simulink model "MainControl_v2"  (R2025a)
settings: Solver=ode45  StartTime=0.0  StopTime=inf  FixedStep=.1  RelTol=1e-3
undefined symbols (not defined in the file or in its folder): CR, DiscIntNeverNeededParam, LF
libraries: instrumentseriallib x3, simulink x1, dspstat3 x1
settings Model: PacingRate=1000  Creator=aceve  LastModifiedBy=diego

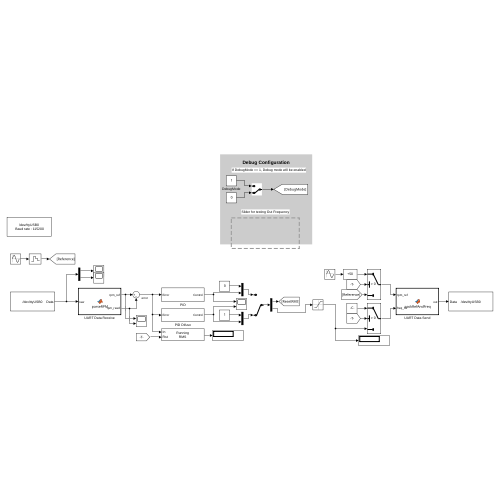
[thumbnail: Simulink's stored preview of the top-level diagram]
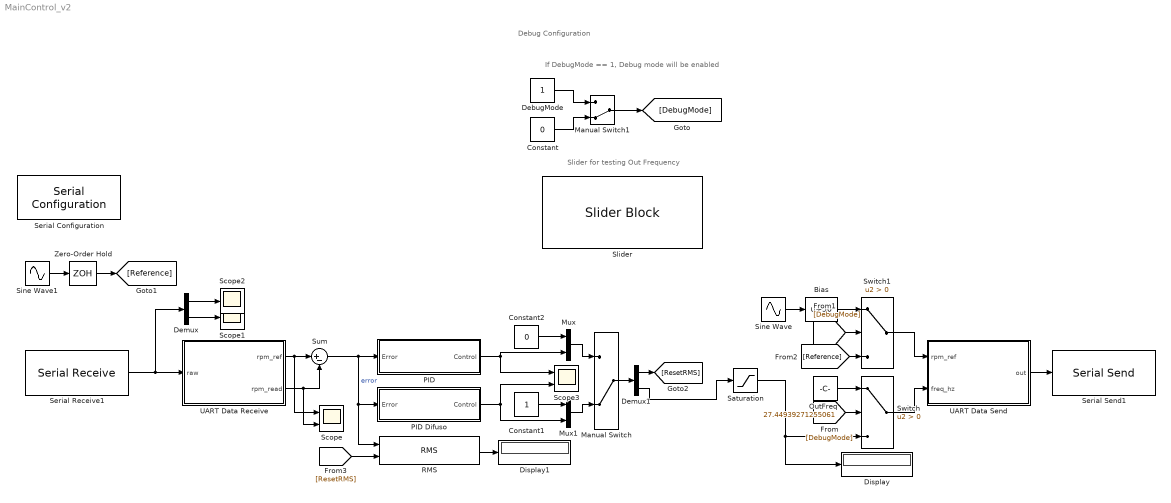
== system MainControl_v2 ==
  note: Debug Configuration
  note: If DebugMode == 1, Debug mode will be enabled
  note: Slider for testing Out Frequency
  Bias : Bias  Bias=50  SaturateOnIntegerOverflow=off
  Constant : Constant  Value=0
  Constant1 : Constant
  Constant2 : Constant  Value=0
  DebugMode : Constant
  Demux : Demux  Outputs=2
  Demux1 : Demux  Outputs=2
  Display : Display
  Display1 : Display
  Manual Switch : ManualSwitch  CurrentSetting=0
  Manual Switch1 : ManualSwitch  CurrentSetting=0
  Mux : Mux  Inputs=2
  Mux1 : Mux  Inputs=2
  OutFreq : Constant  Value=27.44939271255061
  PID : Subsystem
  PID Difuso : Subsystem
  RMS : dspstat3/RMS  run=on  directionMode=Entire input  dimension=1  InputProcessing=Columns as channels (frame based)  reset_popup=Either edge
  Saturation : Saturate  UpperLimit=60  LowerLimit=20
  Scope : Scope  NumInputPorts=2
      settings: ActiveDisplayYMinimum=-88.124999999999986  ActiveDisplayYMaximum=783.125
  Scope1 : Scope
      settings: ActiveDisplayYMinimum=-12.499999999999996  ActiveDisplayYMaximum=112.5
  Scope2 : Scope
      settings: ActiveDisplayYMinimum=-105.87499999999997  ActiveDisplayYMaximum=952.875  DataLoggingVariableName=ScopeData2
  Scope3 : Scope  NumInputPorts=2
      settings: ActiveDisplayYMinimum=-7.4999999999999982  ActiveDisplayYMaximum=67.5  DataLoggingVariableName=ScopeData3
  Serial Configuration : instrumentseriallib/Serial Configuration  Priority=-200000  PortSel=/dev/ttyUSB0  Port=/dev/ttyUSB0  ComPort=/dev/ttyUSB0  BaudRate=115200  DataBits=8  Parity=none  StopBits=1  ByteOrder=little-endian  FlowControl=none  Timeout=10  SimulateUsing=Interpreted execution  BlockInModel=on  aMode=1
  Serial Receive1 : instrumentseriallib/Serial Receive  Priority=1  PortSel=/dev/ttyUSB0  Port=/dev/ttyUSB0  ComPort=/dev/ttyUSB0  DataType=int16  SaveDataType=uint8  ToggleHeader=off  Header=[]  ToggleDataSize=on  DataSize=[2 1]  ToggleTerminator=off  Terminator=CR/LF ('\r\n')  CustomTerminator=[]  InputFormat=Column major  EnableBlockingMode=on  ActionDataUnavailable=Output last received value  ActionWhenDataUnavailable=Output last received value  CustomValue=0  SampleTime=0.01  SimulateUsing=Interpreted execution  BlockInModel=on  aMode=1  LibraryInUse=instrumentlib
  Serial Send1 : instrumentseriallib/Serial Send  Priority=1  PortSel=/dev/ttyUSB0  Port=/dev/ttyUSB0  ComPort=/dev/ttyUSB0  Header=[]  Terminator=<none>  CustomTerminator=[]  EnableBlockingMode=off  SimulateUsing=Interpreted execution  BlockInModel=on  aMode=1
  Sine Wave : Sin  Amplitude=50  SampleTime=0
  Sine Wave1 : Sin  Amplitude=20  Bias=500  Frequency=2  SampleTime=0
  Slider : SliderBlock  ScaleMin=20  ScaleMax=60
  Sum : Sum  Inputs=|+-
  Switch : Switch  Criteria=u2 > Threshold  SaturateOnIntegerOverflow=off  InputSameDT=off
  Switch1 : Switch  Criteria=u2 > Threshold  SaturateOnIntegerOverflow=off  InputSameDT=off
  UART Data Receive : MATLAB Function  TreatAsAtomicUnit=on
  UART Data Send : MATLAB Function  TreatAsAtomicUnit=on
  Zero-Order Hold : ZeroOrderHold  SampleTime=-1
  wires:
  Serial Receive1/1 -> Demux/1, UART Data Receive/1(raw)
  Demux/1 -> Scope2/1
  Demux/2 -> Scope1/1
  Sine Wave/1 -> Bias/1
  UART Data Send/1(out) -> Serial Send1/1
  Switch/1 -> UART Data Send/2(freq_hz)
  [DebugMode] -> Switch/2
  OutFreq/1 -> Switch/1
  Switch1/1 -> UART Data Send/1(rpm_ref)
  Bias/1 -> Switch1/1
  [DebugMode] -> Switch1/2
  Sum/1 -> PID Difuso/1(Error), RMS/1, PID/1(Error)  "error"
  PID Difuso/1(Control) -> Mux1/2, Scope3/2
  PID/1(Control) -> Mux/2, Scope3/1
  UART Data Receive/1(rpm_ref) -> Scope/1, Sum/1
  UART Data Receive/2(rpm_read) -> Scope/2, Sum/2
  Sine Wave1/1 -> Zero-Order Hold/1
  Zero-Order Hold/1 -> [Reference]
  [Reference] -> Switch1/3
  Saturation/1 -> Display/1, Switch/3
  DebugMode/1 -> Manual Switch1/1
  Manual Switch1/1 -> [DebugMode]
  Constant/1 -> Manual Switch1/2
  Constant1/1 -> Mux1/1
  Constant2/1 -> Mux/1
  Mux/1 -> Manual Switch/1
  Mux1/1 -> Manual Switch/2
  Manual Switch/1 -> Demux1/1
  Demux1/2 -> Saturation/1
  Demux1/1 -> [ResetRMS]
  [ResetRMS] -> RMS/2
  RMS/1 -> Display1/1

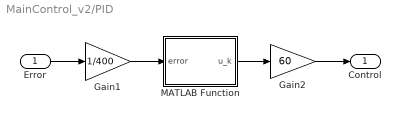
== system MainControl_v2/PID ==
  Error : Inport
  Gain1 : Gain  Gain=1/400
  Gain2 : Gain  Gain=60
  MATLAB Function : MATLAB Function  TreatAsAtomicUnit=on
  Control : Outport
  wires:
  Gain1/1 -> MATLAB Function/1(error)
  MATLAB Function/1(u_k) -> Gain2/1
  Error/1 -> Gain1/1
  Gain2/1 -> Control/1

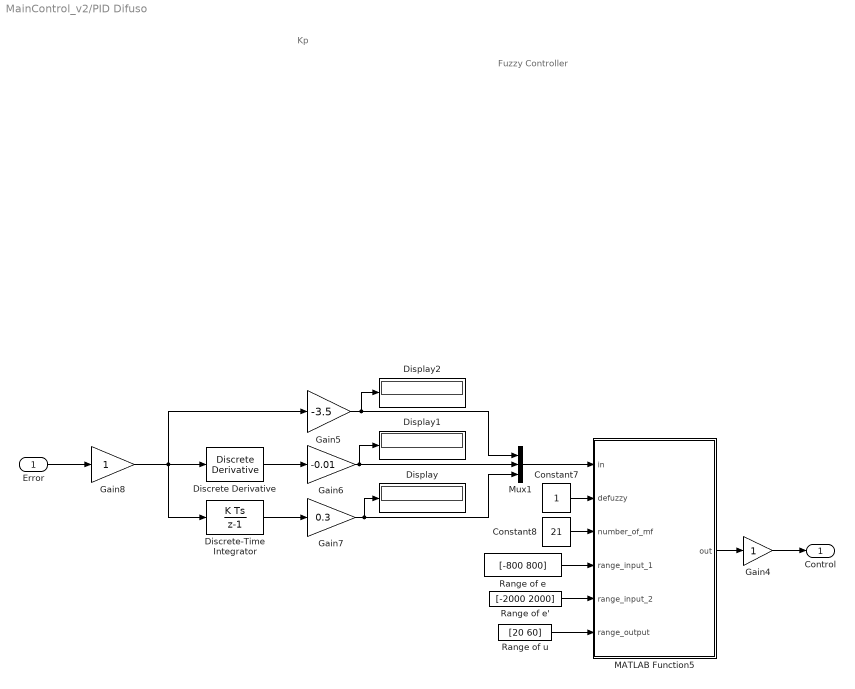
== system MainControl_v2/PID Difuso ==
  note: Fuzzy Controller
  note: Kp
  Error : Inport
  Constant7 : Constant
  Constant8 : Constant  Value=21
  Discrete Derivative : simulink/Discrete/Discrete Derivative  gainval=1.0  ICPrevScaledInput=0.0  OutMin=[]  OutMax=[]  OutDataType=fixdt(1, 16)  OutScaling=2^-10  DoSatur=off
  Discrete-Time Integrator : DiscreteIntegrator  InitialCondition=20  SampleTime=0.01  LimitOutput=on  UpperSaturationLimit=60  LowerSaturationLimit=-60  ICPrevOutput=DiscIntNeverNeededParam  ICPrevScaledInput=DiscIntNeverNeededParam
  Display : Display
  Display1 : Display
  Display2 : Display
  Gain4 : Gain
  Gain5 : Gain  Gain=-3.5
  Gain6 : Gain  Gain=-0.01
  Gain7 : Gain  Gain=0.3
  Gain8 : Gain
  MATLAB Function5 : MATLAB Function  TreatAsAtomicUnit=on
  Mux1 : Mux  Inputs=3
  Range of e : Constant  Value=[-800 800]
  Range of e' : Constant  Value=[-2000 2000]
  Range of u : Constant  Value=[20 60]
  Control : Outport
  wires:
  Gain7/1 -> Mux1/3, Display/1
  Range of e/1 -> MATLAB Function5/4(range_input_1)
  Gain8/1 -> Gain5/1, Discrete-Time Integrator/1, Discrete Derivative/1
  Gain6/1 -> Display1/1, Mux1/2
  MATLAB Function5/1(out) -> Gain4/1
  Constant8/1 -> MATLAB Function5/3(number_of_mf)
  Mux1/1 -> MATLAB Function5/1(in)
  Discrete Derivative/1 -> Gain6/1
  Discrete-Time Integrator/1 -> Gain7/1
  Range of e'/1 -> MATLAB Function5/5(range_input_2)
  Range of u/1 -> MATLAB Function5/6(range_output)
  Constant7/1 -> MATLAB Function5/2(defuzzy)
  Gain5/1 -> Display2/1, Mux1/1
  Gain4/1 -> Control/1
  Error/1 -> Gain8/1

== matlab function MainControl_v2/UART Data Receive ==
  data: rpm_ref output; rpm_read output; raw input
function [rpm_ref, rpm_read] = parseRPM(raw)
%#codegen
% raw: 1x2 uint16 vector received from ESP32
% rpm_read: measured RPM from encoder
% rpm_ref:  reference RPM echoed back from ESP32

rpm_read = double(raw(1));   % first  uint16 from ESP32
rpm_ref  = double(raw(2));   % second uint16 from ESP32
end

== matlab function MainControl_v2/PID Difuso/MATLAB Function5 ==
  data: in input; out output; defuzzy input; number_of_mf input; range_input_1 input; range_input_2 input; range_output input
function out = fcn(in, defuzzy, number_of_mf, range_input_1, range_input_2, range_output)
% CONTROLADOR FUZZY PID (Fuzzy PD + I)
% in: [error_scaled, d_error_scaled, integral_scaled]
% defuzzy: 0 = COG, 1 = CA
% range_input_1/2: [min, max] (Universo para PD)
% range_output: [min, max] (Universo para Salida Final, ej: [6, 54])

% === 1. Preparar divisiones ===
n = number_of_mf;
div1 = linspace(range_input_1(1), range_input_1(2), n); % error
div2 = linspace(range_input_2(1), range_input_2(2), n); % d_error

% El universo de salida del PD difuso. 
% Lo definimos igual que el rango de salida final por simplicidad.
div_out = linspace(range_output(1), range_output(2), n);

% === 2. Calcular membresías de entrada (solo para PD) ===
mu_e = compute_memberships(in(1), div1);
mu_de = compute_memberships(in(2), div2);

% === 3. Definir FAM (PD) ===
FAM = zeros(n, n);
middle_val = (n + 1) / 2;
middle_ij = middle_val*2;
for i = 1:n
    for j = 1:n
        v = middle_val + middle_ij - (i + j);
        if v > n, v = n; end
        if v < 1, v = 1; end
        FAM(i,j) = v;
    end
end

% === 4. Activaciones de reglas (PD) ===
rule_heights = zeros(n,n);
for i = 1:n
    for j = 1:n
        h = min(mu_e(i), mu_de(j));
        rule_heights(i,j) = h;
    end
end
% Max activación por salida
mu_out = zeros(1,n);
for k = 1:n
    % Encuentra todas las reglas (i,j) que tienen la salida k
    mask = (FAM == k);
    if any(mask(:)) % Evita max([]) si una etiqueta de salida no se usa
        mu_out(k) = max(rule_heights(mask));
    else
        mu_out(k) = 0;
    end
end

% === 5. Defuzzificación (Cálculo de la Salida PD) ===
% Usamos un valor central robusto por si den == 0
midL = floor((n+1)/2);
midR = ceil((n+1)/2);
center_val = 0.5*(div_out(midL) + div_out(midR));

fuzzy_pd_out = center_val; % Valor por defecto

if defuzzy == 0
    % --- COG (Centroide) ---
    num = 0; den = 0;
    if n > 1
        step = div_out(2)-div_out(1);
    else
        step = 0; % Evitar error si n=1
    end
    base = 2*step; % base total de cada triángulo
    for k = 1:n
        h = mu_out(k);
        if h > 0
            top_base = (1-h)*base;
            A = h*(base+top_base)/2; % área del trapecio
            num = num + A*div_out(k);
            den = den + A;
        end
    end
    if den > eps
        fuzzy_pd_out = num/den;
    end
else
    % --- CA (Promedio Ponderado) ---
    num = sum(mu_out .* div_out);
    den = sum(mu_out);
    if den > eps
        fuzzy_pd_out = num/den;
    end
end

% === 6. COMBINACIÓN PID (Fuzzy PD + I) ===
% Sumamos la salida difusa PD con la entrada Integral (in(3))
out_unclamped = fuzzy_pd_out + in(3);

% === 7. SATURACIÓN DE SALIDA ===
% Forzamos la salida final a estar dentro del rango [6, 54]
if out_unclamped < range_output(1)
    out = range_output(1); % Mínimo 6V
elseif out_unclamped > range_output(2)
    out = range_output(2); % Máximo 54V
else
    out = out_unclamped;
end

end

% === Función Auxiliar de Membresías ===
function mu = compute_memberships(x, div)
n = length(div);
mu = zeros(1,n);
if x <= div(1)
    mu(1) = 1; return
elseif x >= div(end)
    mu(end) = 1; return
end
for i = 1:n-1
    x1 = div(i); x2 = div(i+1);
    den = x2 - x1;
    if den == 0, den = eps; end % Evitar división por cero
    
    if x >= x1 && x <= x2
        mu(i) = (x2 - x)/den;
        mu(i+1) = (x - x1)/den;
        return
    end
end
end

== matlab function MainControl_v2/UART Data Send ==
  data: rpm_ref input; freq_hz input; out output
function out = packRefAndFreq(rpm_ref, freq_hz)

freq_u16 = uint16(freq_hz);

rpm_u16 = uint16(rpm_ref);

out = uint16([rpm_u16, freq_u16]);
end

== matlab function MainControl_v2/PID/MATLAB Function ==
  data: error input; u_k output
function u_k = PID(error)
% Esta función implementa el controlador PID discreto del código de Arduino.
% ENTRADA:
%   error: El error actual e(k) = (referencia - medida)
% SALIDA:
%   u_k: La señal de control saturada (entre 0.0 y 1.0)

% ===== Parámetros del Controlador (iguales a los de Arduino) =====
Kc = 0.12;
Ti = 0.05;
Td = 0.005;
N = 100;
Ts_s = 0.01; % Periodo de muestreo en segundos (20 ms)

% ===== Variables de Estado (persisten entre llamadas) =====
% Se declaran como 'persistent' para que guarden su valor,
% igual que las variables globales en Arduino.
persistent error_prev integral_prev derivative_prev

% ===== Inicialización en la primera ejecución =====
% La primera vez que se llama a la función, las variables están vacías.
if isempty(error_prev)
    error_prev = 0.0;
    integral_prev = 0.0;
    derivative_prev = 0.0;
end

% ================================================================
% ===== LÓGICA DE CONTROL PID (Traducción directa de C++) ========
% ================================================================

% 2. Calcular término Proporcional: p(k) = Kc * e(k)
p_k = Kc * error;

% 3. Calcular término Integral: i(k) = i(k-1) + (h*Kc/Ti) * e(k)
i_k = integral_prev + (Kc * Ts_s / Ti) * error;

% 4. Calcular término Derivativo: d(k) = c1*d(k-1) + c2*e(k) - c2*e(k-1)
c1 = 1.0 / (1.0 + Ts_s * N);
c2 = (Kc * Td * N) / (1.0 + Ts_s * N);
d_k = c1 * derivative_prev + c2 * (error - error_prev);

% 5. Calcular la salida de control total: u(k) = p(k) + i(k) + d(k)
u_k_total = p_k + i_k + d_k;

% --- Saturación y Anti-Windup ---
u_k_saturado = u_k_total;
if u_k_saturado > 1.0
    u_k_saturado = 1.0;
end
if u_k_saturado < 0.0
    u_k_saturado = 0.0;
end

% --- Actualización de estados para la siguiente iteración ---
% Anti-Windup: Actualizar el término integral solo si no hay saturación
if u_k_total == u_k_saturado
    integral_prev = i_k;
end
derivative_prev = d_k;
error_prev = error;

% Asignar la salida final de la función
u_k = u_k_saturado;

end
